simulink model "Osc_sec"  (R2020a)
settings: Solver=VariableStepAuto  StartTime=0.0  StopTime=1/f_s  FixedStep=fixed_step_size  RelTol=1e-3
values from neighbouring files (symbols this model uses):
  C_p = (12 / N_p) ^ 2 * 16e-12    [TLNPC_Brute_force_update.m]
  C_r = 60e-12    (= 6e-11)    [TLNPC_Brute_force_update.m]
  C_s = (12 / N_s) ^ 2 * 10e-12    [TLNPC_Brute_force_update.m]
  L_ac_1 = L_ac * L_ac_ratio / (L_ac_ratio + 1)    [TLNPC_Brute_force_update.m]
  L_ac_2 = L_ac * 1 / (L_ac_ratio + 1)    [TLNPC_Brute_force_update.m]
  L_kp = L_kp_T * N_p    [TLNPC_Brute_force_update.m]
  L_ks = L_ks_T * N_s    [TLNPC_Brute_force_update.m]
  Lac_s = 100e-9    (= 1e-07)    [TLNPC_Brute_force_update.m]
  N_p = Para_ana(p,9)    [TLNPC_Brute_force_update.m]
  N_s = N_p / T_ratio    [TLNPC_Brute_force_update.m]
  R_Lac_1 = R_T_Lac * N_T_Lac_1    [TLNPC_Brute_force_update.m]
  R_Lac_2 = R_T_Lac * N_T_Lac_2    [TLNPC_Brute_force_update.m]
  R_lkp = R_T_p * N_p    [TLNPC_Brute_force_update.m]
  R_lks = R_T_s * N_s    [TLNPC_Brute_force_update.m]
  V_in = 1200    [TLNPC_Brute_force_update.m]
libraries: powerlib x13
settings Model: Creator=yudxiao  LastModifiedBy=yudxiao
settings DataIOCC: ExternalInput=getinputstruct(op_snapshot1)  InitialState=getstatestruct(op_snapshot1)  DSMLogging=off
settings SFSimCC: CustomCodeUndefinedFunction=UseInterfaceOnly

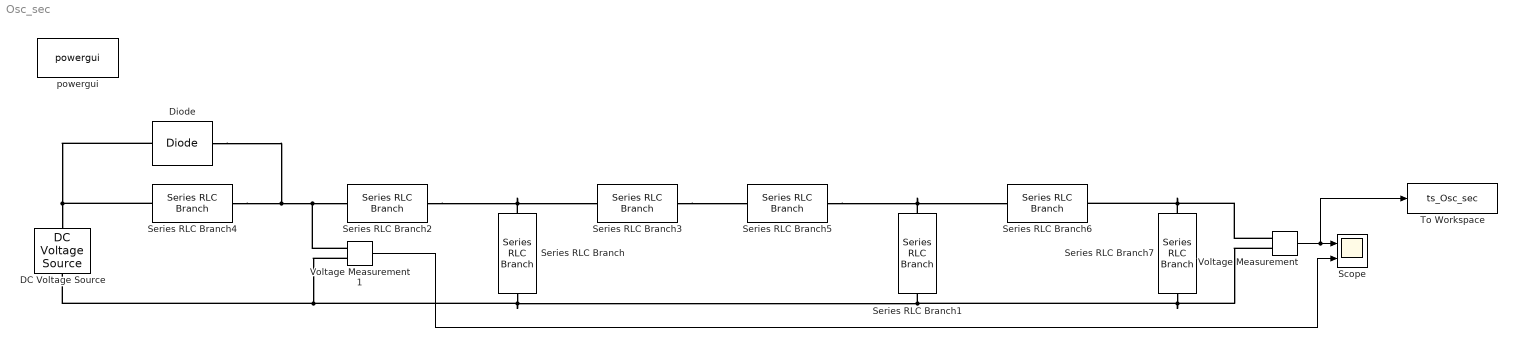
== system Osc_sec ==
  DC Voltage Source : powerlib/Electrical Sources/DC Voltage Source  Amplitude=V_in/2  Measurements=None
  Diode : powerlib/Power Electronics/Diode  Ron=0  Lon=0  Vf=0  IC=0  UseSnubber=0  Rs=inf  Cs=0  Measurements=off
  Scope : Scope  NumInputPorts=2
  Series RLC Branch : powerlib/Elements/Series RLC Branch  LConnTagsString=__new0  RConnTagsString=__new0  BranchType=C  Resistance=1  Inductance=1e-3  SetiL0=off  InitialCurrent=0  Capacitance=C_p  Setx0=on  InitialVoltage=0  Measurements=None
  Series RLC Branch1 : powerlib/Elements/Series RLC Branch  LConnTagsString=__new0  RConnTagsString=__new0  BranchType=C  Resistance=1  Inductance=1e-3  SetiL0=off  InitialCurrent=0  Capacitance=C_s/((N_p/N_s)*(N_p/N_s))  Setx0=on  InitialVoltage=0  Measurements=None
  Series RLC Branch2 : powerlib/Elements/Series RLC Branch  LConnTagsString=__new0  RConnTagsString=__new0  BranchType=RL  Resistance=R_Lac_2  Inductance=L_ac_2  SetiL0=off  InitialCurrent=I_2  Capacitance=1e-6  Setx0=off  InitialVoltage=0  Measurements=None
  Series RLC Branch3 : powerlib/Elements/Series RLC Branch  LConnTagsString=__new0  RConnTagsString=__new0  BranchType=RL  Resistance=R_lkp  Inductance=L_kp  SetiL0=off  InitialCurrent=0  Capacitance=1e-6  Setx0=off  InitialVoltage=0  Measurements=None
  Series RLC Branch4 : powerlib/Elements/Series RLC Branch  LConnTagsString=__new0  RConnTagsString=__new0  BranchType=RL  Resistance=R_Lac_1  Inductance=L_ac_1  SetiL0=on  InitialCurrent=I_2  Capacitance=1e-6  Setx0=off  InitialVoltage=0  Measurements=None
  Series RLC Branch5 : powerlib/Elements/Series RLC Branch  LConnTagsString=__new0  RConnTagsString=__new0  BranchType=RL  Resistance=R_lks*(N_p/N_s)*(N_p/N_s)  Inductance=L_ks*(N_p/N_s)*(N_p/N_s)  SetiL0=on  InitialCurrent=0  Capacitance=1e-6  Setx0=off  InitialVoltage=0  Measurements=None
  Series RLC Branch6 : powerlib/Elements/Series RLC Branch  LConnTagsString=__new0  RConnTagsString=__new0  BranchType=L  Resistance=1  Inductance=Lac_s*(N_p/N_s)*(N_p/N_s)  SetiL0=on  InitialCurrent=0  Capacitance=1e-6  Setx0=off  InitialVoltage=0  Measurements=None
  Series RLC Branch7 : powerlib/Elements/Series RLC Branch  LConnTagsString=__new0  RConnTagsString=__new0  BranchType=C  Resistance=1  Inductance=1e-3  SetiL0=off  InitialCurrent=0  Capacitance=C_r/((N_p/N_s)*(N_p/N_s))  Setx0=on  InitialVoltage=0  Measurements=None
  To Workspace : ToWorkspace  VariableName=ts_Osc_sec  SaveFormat=Timeseries  SampleTime=-1
  Voltage Measurement : powerlib/Measurements/Voltage Measurement  PhasorSimulation=off  OutputType=Complex  PSBequivalent=0
  Voltage Measurement1 : powerlib/Measurements/Voltage Measurement  PhasorSimulation=off  OutputType=Complex  PSBequivalent=0
  powergui : powerlib/powergui  Priority=1  SimulationMode=Continuous  SampleTime=50e-6  frequency=60  Iterations=50  frequencyindice=0  Pbase=100e6  ErrMax=1e-4  UnitsV=kV  UnitsW=MW  buscounter=0  FunctionMessages=off  echomessages=off  EnableUseOfTLC=off  CurrentSourceSwitches=off  DisableSnubberDevices=off  DisableRonSwitches=off  DisableVfSwitches=off  DisplayEquations=off  AutomaticDiscreteSolvers=off  SolverType=Tustin/Backward Euler (TBE)  Interpol=off  ExternalGateDelay=off  methode=off  Ts=100  x0status=blocks  SPID=on  SwTol=0  HookPort=off  NonlinearTolerance=0  nMaxIteration=15  ContinueOnMaxIteration=off  RestoreLinks=warning  ResistiveCurrentMeasurement=off  Frange=[0:2:500]  Ylog=off  Xlog=on  ShowGrid=off  save=off  variable=ZData  structure=0  ZoomFFT=off  StartTime=0.0  cycles=1  DisplayStyle=1  fundamental=60  FreqAxis=off  MaxFrequency=1000  frequencyindicesteady=1  RmsSteady=1  display=off
  wires:
  Voltage Measurement/1 -> To Workspace/1, Scope/1
  Voltage Measurement1/1 -> Scope/2
  connections:
  Voltage Measurement/LConn2 -- Series RLC Branch7/RConn1 -- Series RLC Branch1/RConn1 -- Series RLC Branch/RConn1 -- Voltage Measurement1/LConn2 -- DC Voltage Source/LConn1
  Series RLC Branch4/RConn1 -- Voltage Measurement1/LConn1 -- Series RLC Branch2/LConn1 -- Diode/LConn1
  Series RLC Branch2/RConn1 -- Series RLC Branch3/LConn1 -- Series RLC Branch/LConn1
  Series RLC Branch3/RConn1 -- Series RLC Branch5/LConn1
  Diode/RConn1 -- Series RLC Branch4/LConn1 -- DC Voltage Source/RConn1
  Series RLC Branch1/LConn1 -- Series RLC Branch6/LConn1 -- Series RLC Branch5/RConn1
  Series RLC Branch7/LConn1 -- Series RLC Branch6/RConn1 -- Voltage Measurement/LConn1
